simulink model "DragBlock_V1"  (R2022a)
settings: Solver=VariableStepAuto  StartTime=0.0  StopTime=10.0  RelTol=1e-3
settings Model: Creator=antonisioannou  LastModifiedBy=antonisioannou

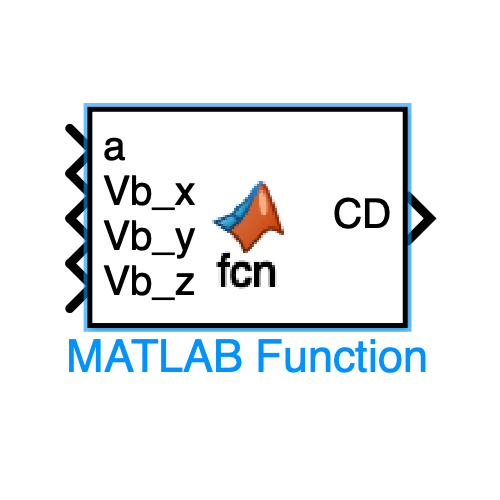
[thumbnail: Simulink's stored preview of the top-level diagram]
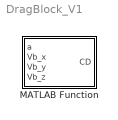
== system DragBlock_V1 ==
  MATLAB Function : MATLAB Function  TreatAsAtomicUnit=on

== matlab function DragBlock_V1/MATLAB Function ==
  data: a input; CD output; Vb_x input; Vb_y input; Vb_z input
function CD = fcn(a, Vb_x, Vb_y, Vb_z)
% Dimensions
b= ; %Distance from fin-tip to fin-tip
d= ; %Body diameters
N_f= ; % Number of fins
C_R= ;   %Root fin chord
S_f=C_R*N_F*(b-d)/2 %Fin Surface Area 

%Reynolds Number Calc.
v=(Vb_x^2+Vb_y^2+Vb_z^2)^0.5;
Re=rho*v*L/mu;

% Laminar Boundary Layer -- Use Blasius Solution (Aero3)
Cf_lam=0.664*(Re)^(-1/2);

% Turbulent Boundart Layer -- Use Emprical Solution (Aero3)
Cf_turb=0.0576*(Re)^(-1/5);

% Nose Cone & Body Tube drag coeff.

CD_noseandbody=1.02*Cf_turb*S_BT/A_BT*(1+1.5/L_d^(3/2));

%Fin Drag coeff.    

CD_Fin=2*Cf_lam*(1+2*t/c_mean)*S_f/A_BT;

%Interference Drag coeff.

CD_I=Cf_turb*(1+2*t/c_mean)*d*N_f*C_R/S_BT;
